simulink model "M_QAM"  (R2017a)
settings: Solver=VariableStepDiscrete  StartTime=0.0  StopTime=100  RelTol=1e-3
libraries: simulink_extras x2, commdigbbndam3 x2, commchan3 x1, commsink2 x1, commrandsrc3 x1
settings Model: Creator=JBlanco  LastModifiedBy=JBlanco

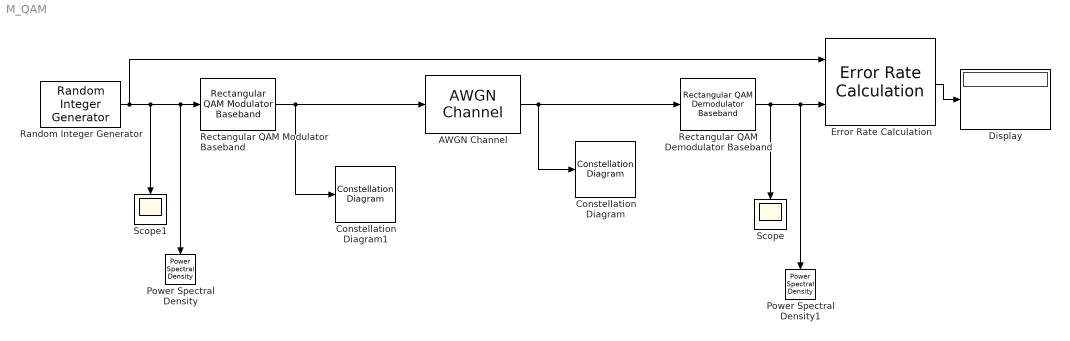
== system M_QAM ==
  AWGN Channel : commchan3/AWGN Channel  InputProcessing=Inherited (this choice will be removed - see release notes)  seed=37  noiseMode="Signal to noise ratio  (Eb/No)"  EbNodB=10  EsNodB=10  SNRdB=10  bitsPerSym=1  Ps=1  Tsym=0.1  variance=1
  Constellation Diagram : ConstellationDiagram
  Constellation Diagram1 : ConstellationDiagram
  Display : Display
  Error Rate Calculation : commsink2/Error Rate Calculation  N=0  st_delay=0  cp_mode=Entire frame  subframe=[]  PMode=Port  WsName=ErrorVec  RsMode2=off  stop=off  numErr=100  maxBits=1e6
  Power Spectral Density : simulink_extras/Additional Sinks/Power Spectral Density  npts=128  fftpts=512  HowOften=64  sampleT=0.1
      settings: SourceProductName=Simulink  SourceProductBaseCode=SL
  Power Spectral Density1 : simulink_extras/Additional Sinks/Power Spectral Density  npts=128  fftpts=512  HowOften=64  sampleT=0.1
      settings: SourceProductName=Simulink  SourceProductBaseCode=SL
  Random Integer Generator : commrandsrc3/Random Integer Generator  SetSize=64  SeedSource=Parameter  Seed=37  SampleTime=.1  SamplesPerFrame=1  OutputDataType=double  SimulateUsing=Interpreted execution
  Rectangular QAM Demodulator Baseband : commdigbbndam3/Rectangular QAM Demodulator Baseband  M=64  OutType=Integer  DecType=Hard decision  VarSource=Dialog  Variance=1  Dec=Binary  Mapping=[0:15]  PowType=Peak Power  MinDist=2  AvgPow=1  PeakPow=1  Ph=0  outDtype1=Inherit via internal rule  outDtype2=Inherit via internal rule  derotateFactorWordLen=16  derotateFactorDataTypeStr=Inherit: Same word length as input  derotateFactorLastDataTypeStr=Inherit: Same word length as input  denormFactorWordLen=16  denormFactorDataTypeStr=Inherit: Same word length as input  denormFactorLastDataTypeStr=Inherit: Same word length as input  prodOutWordLen=32  prodOutOverflowMode=Wrap  prodOutRoundingMode=Floor  prodOutOvFlMode=off  prodOutOvFlModeLastStrValue=off  sumWordLen=32
  Rectangular QAM Modulator Baseband : commdigbbndam3/Rectangular QAM Modulator Baseband  M=64  InType=Integer  Enc=Binary  Mapping=[0:15]  PowType=Peak Power  MinDist=2  AvgPow=1  PeakPow=1  Ph=0  outDtype=double  outWordLen=16  outUDDataType=sfix(16)  outFracLenMode=Best precision  outFracLen=15  outDataTypeStr=double  outLastDataTypeStr=double
  Scope : Scope
  Scope1 : Scope
  wires:
  Random Integer Generator/1 -> Error Rate Calculation/1, Rectangular QAM Modulator Baseband/1, Power Spectral Density/1, Scope1/1
  AWGN Channel/1 -> Rectangular QAM Demodulator Baseband/1, Constellation Diagram/1
  Rectangular QAM Modulator Baseband/1 -> AWGN Channel/1, Constellation Diagram1/1
  Rectangular QAM Demodulator Baseband/1 -> Power Spectral Density1/1, Error Rate Calculation/2, Scope/1
  Error Rate Calculation/1 -> Display/1
